simulink model "satellite_propagator"  (R2025a)
settings: Solver=ode45  StartTime=0.0  StopTime=3600  RelTol=1e-3
settings Model: Creator=ako  LastModifiedBy=ako

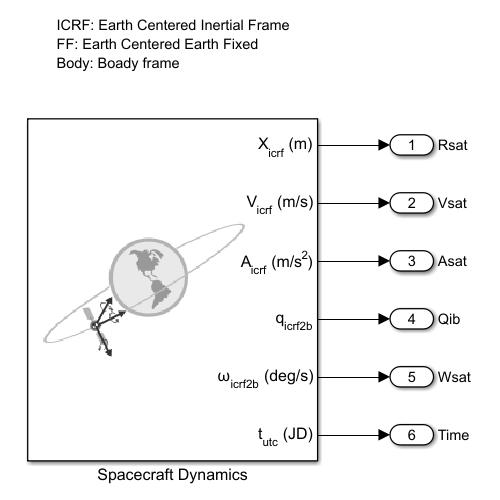
[thumbnail: Simulink's stored preview of the top-level diagram]
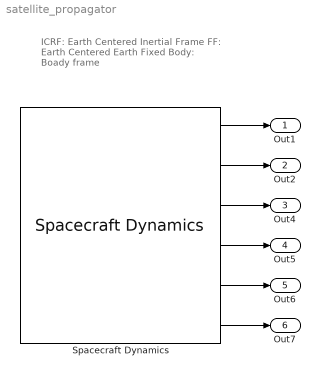
== system satellite_propagator ==
  note: ICRF: Earth Centered Inertial Frame
      | FF: Earth Centered Earth Fixed
      | Body: Boady frame
  Spacecraft Dynamics : SpacecraftDynamics  forcesIn=off  momentsIn=off  outputAccel=on  startDate=startTimeJD  semiMajorAxis=a  eccentricity=e  inclination=inclination  raan=raan  argPeriapsis=aop  trueAnomaly=ta  attitude=q0  attitudeRate=w0  useGravGrad=off  gravityModel=Point-mass  useEOPs=off
  Out1 : Outport  SignalName=Rsat
  Out2 : Outport  Port=2  SignalName=Vsat
  Out4 : Outport  Port=3  SignalName=Asat
  Out5 : Outport  Port=4  SignalName=Qib
  Out6 : Outport  Port=5  SignalName=Wsat
  Out7 : Outport  Port=6  SignalName=Time
  wires:
  Spacecraft Dynamics/1 -> Out1/1
  Spacecraft Dynamics/2 -> Out2/1
  Spacecraft Dynamics/3 -> Out4/1
  Spacecraft Dynamics/4 -> Out5/1
  Spacecraft Dynamics/5 -> Out6/1
  Spacecraft Dynamics/6 -> Out7/1
